simulink model "SIM_nominal"  (R2023b)
settings: Solver=VariableStepAuto  StartTime=0.0  StopTime=1200  RelTol=1e-3
values from neighbouring files (symbols this model uses):
  Ts = 3    [NMPC_FOUR_TANKS.m]
  u0 = [55;75]    [NMPC_FOUR_TANKS.m]
libraries: mpclib x1
settings Model: Creator=akeebismail  LastModifiedBy=akeebismail

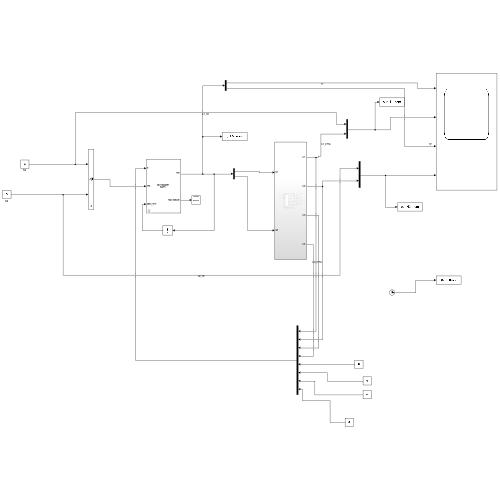
[thumbnail: Simulink's stored preview of the top-level diagram]
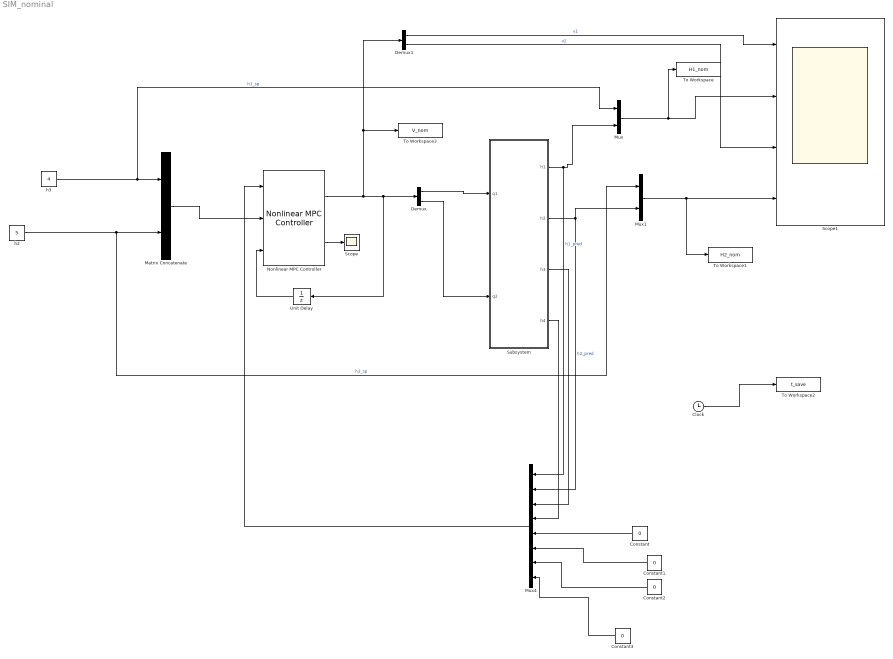
== system SIM_nominal ==
  Clock : Clock
  Constant{,1..3} (4 alike) : Constant  Value=0
  Demux : Demux  Outputs=2
  Demux1 : Demux  Outputs=2
  Matrix Concatenate : Concatenate  Mode=Multidimensional array  ConcatenateDimension=2
  Mux : Mux  Inputs=2
  Mux1 : Mux  Inputs=2
  Mux4 : Mux  Inputs=8
  Nonlinear MPC Controller : mpclib/Nonlinear MPC Controller  nlmpcobj=nlobj  UseObjectTs=on  UseMEX=off  md_enabled=off  mvtarget_enabled=off  param_enabled=off  cost_enabled=off  mvseq_enabled=off  stateseq_enabled=off  ovseq_enabled=off  slack_enabled=off  status_enabled=on  ov_min=off  ov_max=off  mv_min=off  mv_max=off  mvrate_min=off  mvrate_max=off  state_min=off  state_max=off  ov_weight=off  mv_weight=off  mvrate_weight=off  ecr_weight=off  nlp_initialize=off
  Scope : Scope
  Scope1 : Scope  NumInputPorts=4
  Subsystem : Subsystem
  To Workspace : ToWorkspace  VariableName=H1_nom  SaveFormat=Timeseries  SampleTime=Ts
  To Workspace1 : ToWorkspace  VariableName=H2_nom  SaveFormat=Timeseries  SampleTime=Ts
  To Workspace2 : ToWorkspace  VariableName=t_save  SaveFormat=Timeseries  SampleTime=Ts
  To Workspace3 : ToWorkspace  VariableName=V_nom  SaveFormat=Timeseries  SampleTime=Ts
  Unit Delay : UnitDelay  InitialCondition=u0  SampleTime=-1  HasFrameUpgradeWarning=on
  h2 : Constant  Value=5
  h3 : Constant  Value=4
  wires:
  Subsystem/2(h2) -> Mux4/2, Mux1/2  "h2_pred"
  Nonlinear MPC Controller/2 -> Scope/1
  Demux/2 -> Subsystem/2(q2)
  h2/1 -> Matrix Concatenate/2, Mux1/1  "h2_sp"
  h3/1 -> Mux/1, Matrix Concatenate/1  "h1_sp"
  Unit Delay/1 -> Nonlinear MPC Controller/3
  Demux1/1 -> Scope1/1  "v1"
  Nonlinear MPC Controller/1 -> To Workspace3/1, Demux1/1, Unit Delay/1, Demux/1
  Subsystem/1(h1) -> Mux/2, Mux4/1  "h1_pred"
  Mux/1 -> To Workspace/1, Scope1/2
  Mux1/1 -> To Workspace1/1, Scope1/4
  Demux1/2 -> Scope1/3  "v2"
  Matrix Concatenate/1 -> Nonlinear MPC Controller/2
  Demux/1 -> Subsystem/1(q1)
  Subsystem/3(h3) -> Mux4/3
  Subsystem/4(h4) -> Mux4/4
  Constant/1 -> Mux4/5
  Constant1/1 -> Mux4/6
  Constant2/1 -> Mux4/7
  Constant3/1 -> Mux4/8
  Mux4/1 -> Nonlinear MPC Controller/1
  Clock/1 -> To Workspace2/1

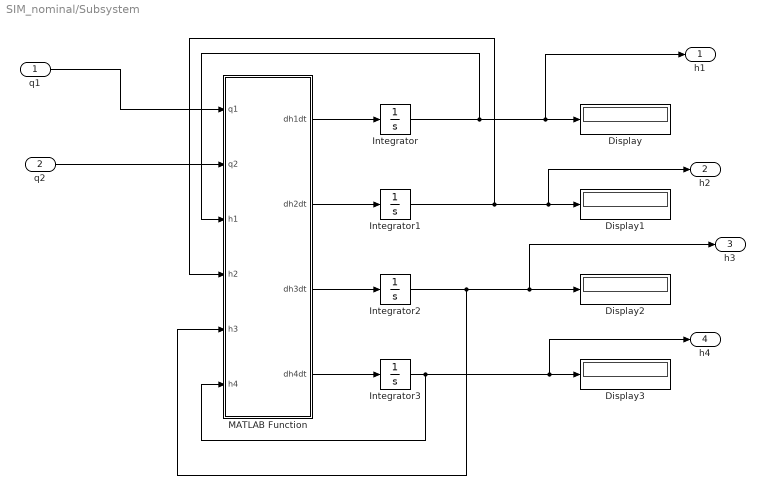
== system SIM_nominal/Subsystem ==
  q1 : Inport
  q2 : Inport  Port=2
  Display{,1..3} (4 alike) : Display
  Integrator{,1..3} (4 alike) : Integrator
  MATLAB Function : MATLAB Function  TreatAsAtomicUnit=on
  h1 : Outport
  h2 : Outport  Port=2
  h3 : Outport  Port=3
  h4 : Outport  Port=4
  wires:
  Integrator1/1 -> MATLAB Function/4(h2), h2/1, Display1/1
  q2/1 -> MATLAB Function/2(q2)
  Integrator3/1 -> MATLAB Function/6(h4), h4/1, Display3/1
  q1/1 -> MATLAB Function/1(q1)
  Integrator2/1 -> MATLAB Function/5(h3), h3/1, Display2/1
  MATLAB Function/2(dh2dt) -> Integrator1/1
  MATLAB Function/1(dh1dt) -> Integrator/1
  MATLAB Function/4(dh4dt) -> Integrator3/1
  MATLAB Function/3(dh3dt) -> Integrator2/1
  Integrator/1 -> MATLAB Function/3(h1), h1/1, Display/1

== matlab function SIM_nominal/Subsystem/MATLAB Function ==
  data: q1 input; dh1dt output; q2 input; h1 input; h2 input; h3 input; h4 input; dh2dt output; dh3dt output; dh4dt output
function [dh1dt,dh2dt,dh3dt,dh4dt] = fcn(q1,q2,h1,h2,h3,h4)
values = {0.97,0.42,0.74,0.426,0.8542,0.7126,0.7722,0.5149,35,35,39,39,981,0.23,0.19};
[a1,a3,a2,a4,alpha1,alpha3,alpha2,alpha4,A1,A3,A2,A4,g,gamma1,gamma2] = values{:};

%F = k1 * v1;
%F2 = k2 * v2;

    dh1dt = -(a1*alpha1/A1) * sqrt(2 * g * h1) + (a3*alpha3/A1) * sqrt(2 * g * h3) + (gamma1 * q1) / A1;
    dh2dt = -(a2*alpha2/A2) * sqrt(2 * g * h2) + (a4*alpha4/A2) * sqrt(2 * g * h4) + (gamma2 * q2) / A2;
    dh3dt = -(a3*alpha3/A3) * sqrt(2 * g * h3) + ((1 - gamma2) * q2) / A3;
    dh4dt = -(a4*alpha4/A4) * sqrt(2 * g * h4) + ((1 - gamma1) * q1) / A4;

end
